simulink model "CIC_FILTER"  (R2018b)
settings: Solver=VariableStepAuto  StartTime=0.0  StopTime=10.0  RelTol=1e-3
libraries: simulink x2, dspsrcs4 x2, hdlsllib x1
settings Model: Creator=MrGoshak  LastModifiedBy=MrGoshak

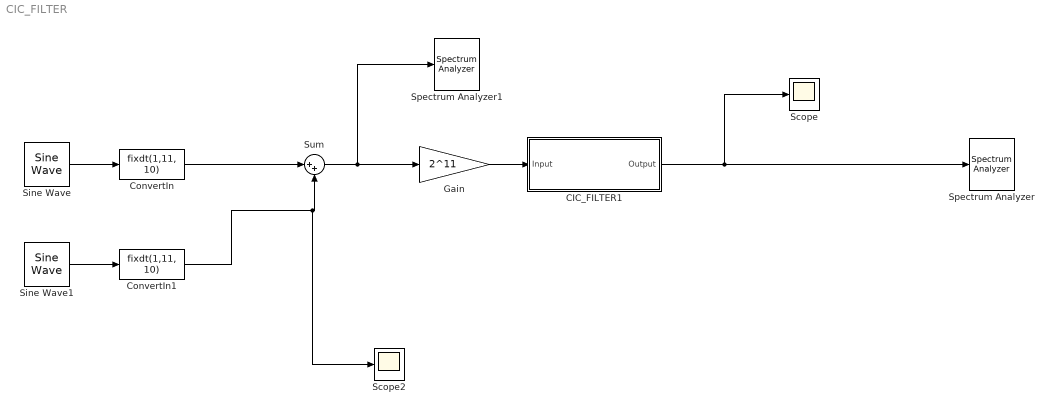
== system CIC_FILTER ==
  CIC_FILTER1 : Subsystem  Tag=FilterWizardSubSystem
      settings: ErrorFcn=dspFilterRealizedInBasicElemsAlgLoopErrFcnCallback
  ConvertIn : DataTypeConversion  OutDataTypeStr=fixdt(1,11, 10)  RndMeth=Nearest  SaturateOnIntegerOverflow=on
  ConvertIn1 : DataTypeConversion  OutDataTypeStr=fixdt(1,11, 10)  RndMeth=Nearest  SaturateOnIntegerOverflow=on
  Gain : Gain  Gain=2^11  OutDataTypeStr=fixdt(1, 16, 0)
  Scope : Scope
  Scope2 : Scope
  Sine Wave : dspsrcs4/Sine Wave  Amplitude=1/2  Frequency=10000  Phase=0  SampleMode=Discrete  OutComplex=Real  CompMethod=Trigonometric fcn  TableSize=Speed  SampleTime=1/500000  SamplesPerFrame=1  ResetState=Restart at time zero  OutputFrames=off  dataType=double  wordLen=15  udDataType=sfix(16)  fracBitsMode=User-defined  numFracBits=0  OutDataTypeStr=double  LastOutDataTypeStr=double
  Sine Wave1 : dspsrcs4/Sine Wave  Amplitude=1/2  Frequency=60000  Phase=0  SampleMode=Discrete  OutComplex=Real  CompMethod=Trigonometric fcn  TableSize=Speed  SampleTime=1/500000  SamplesPerFrame=1  ResetState=Restart at time zero  OutputFrames=off  dataType=double  wordLen=16  udDataType=sfix(16)  fracBitsMode=Best precision  numFracBits=15  OutDataTypeStr=double  LastOutDataTypeStr=double
  Spectrum Analyzer : SpectrumAnalyzer
  Spectrum Analyzer1 : SpectrumAnalyzer
  Sum : Sum  Inputs=|++  OutDataTypeStr=fixdt(1,12, 11)  SaturateOnIntegerOverflow=on  InputSameDT=on
  wires:
  Sine Wave/1 -> ConvertIn/1
  ConvertIn/1 -> Sum/1
  ConvertIn1/1 -> Scope2/1, Sum/2
  Sine Wave1/1 -> ConvertIn1/1
  Sum/1 -> Gain/1, Spectrum Analyzer1/1
  CIC_FILTER1/1(Output) -> Scope/1, Spectrum Analyzer/1
  Gain/1 -> CIC_FILTER1/1(Input)

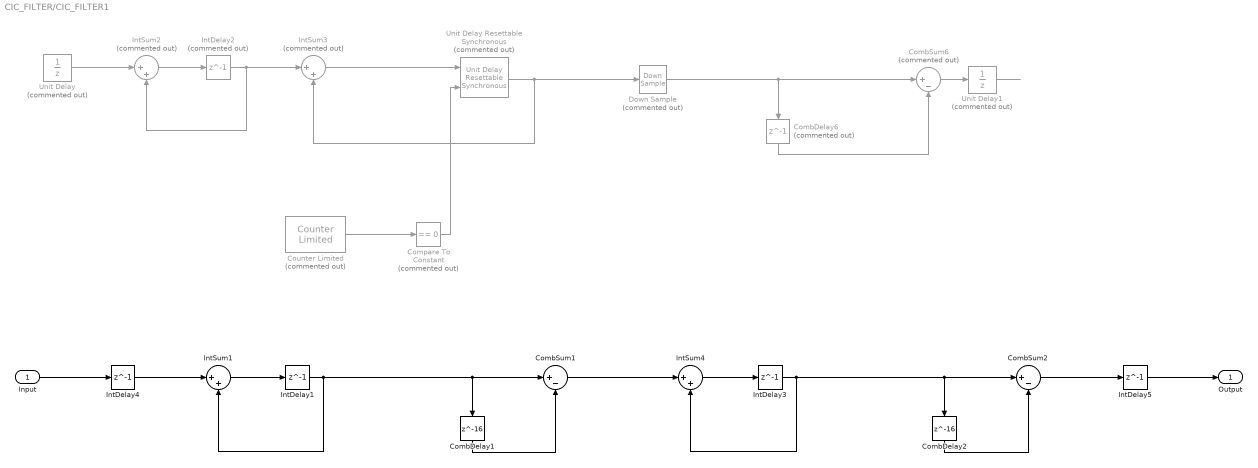
== system CIC_FILTER/CIC_FILTER1 ==
  Input : Inport
  CombDelay1 : Delay  DelayLength=16  InitialCondition=0
  CombDelay2 : Delay  DelayLength=16  InitialCondition=0
  CombDelay6 : Delay  Commented=on  DelayLength=1  InitialCondition=0
  CombSum1 : Sum  Inputs=|+-  AccumDataTypeStr=fixdt(1,20,0)  OutDataTypeStr=fixdt(1,20,0)
  CombSum2 : Sum  Inputs=|+-  AccumDataTypeStr=fixdt(1,20,0)  OutDataTypeStr=fixdt(1,20,0)
  CombSum6 : Sum  Commented=on  Inputs=|+-  AccumDataTypeStr=fixdt(1,18,0)  OutDataTypeStr=fixdt(1,18,0)
  Compare To Constant : simulink/Logic and Bit Operations/Compare To Constant  Commented=on  relop===  const=0  OutDataTypeStr=boolean
  Counter Limited : simulink/Sources/Counter Limited  Commented=on  uplimit=1  tsamp=1/500000
  Down Sample : DownSample  Commented=on  RateOptions=Allow multirate processing
  IntDelay{1,3..5} (4 alike) : Delay  DelayLength=1  InitialCondition=0
  IntDelay2 : Delay  Commented=on  DelayLength=1  InitialCondition=0
  IntSum1 : Sum  Inputs=|++  AccumDataTypeStr=fixdt(1,20,0)  OutDataTypeStr=fixdt(1,20,0)
  IntSum2 : Sum  Commented=on  Inputs=|++  AccumDataTypeStr=fixdt(1,18,0)  OutDataTypeStr=fixdt(1,18,0)
  IntSum3 : Sum  Commented=on  Inputs=|++  AccumDataTypeStr=fixdt(1,18,0)  OutDataTypeStr=fixdt(1,18,0)
  IntSum4 : Sum  Inputs=|++  AccumDataTypeStr=fixdt(1,20,0)  OutDataTypeStr=fixdt(1,20,0)
  Unit Delay : UnitDelay  Commented=on  SampleTime=-1
  Unit Delay Resettable Synchronous : hdlsllib/Discrete/Unit Delay Resettable Synchronous  Commented=on  InitialCondition=0.0  SampleTime=-1
      settings: SourceProductName=HDL Coder  SourceProductBaseCode=HD
  Unit Delay1 : UnitDelay  Commented=on  SampleTime=-1
  Output : Outport
  wires:
  ? -> Unit Delay/1
  IntSum2/1 -> IntDelay2/1
  IntDelay2/1 -> IntSum2/2, IntSum3/1
  IntSum3/1 -> Unit Delay Resettable Synchronous/1
  Down Sample/1 -> CombSum6/1, CombDelay6/1
  CombDelay6/1 -> CombSum6/2
  CombSum6/1 -> Unit Delay1/1
  Counter Limited/1 -> Compare To Constant/1
  Compare To Constant/1 -> Unit Delay Resettable Synchronous/2
  Unit Delay Resettable Synchronous/1 -> IntSum3/2, Down Sample/1
  Unit Delay/1 -> IntSum2/1
  Unit Delay1/1 -> ?
  Input/1 -> IntDelay4/1
  IntDelay1/1 -> CombSum1/1, CombDelay1/1, IntSum1/2
  IntSum1/1 -> IntDelay1/1
  CombDelay1/1 -> CombSum1/2
  IntSum4/1 -> IntDelay3/1
  CombSum1/1 -> IntSum4/1
  IntDelay3/1 -> CombSum2/1, CombDelay2/1, IntSum4/2
  CombDelay2/1 -> CombSum2/2
  CombSum2/1 -> IntDelay5/1
  IntDelay4/1 -> IntSum1/1
  IntDelay5/1 -> Output/1
